simulink model "w3_warplab_trigger_proc"  (Simulink 7.7)
settings: Solver=ode45  StartTime=0.0  StopTime=60  RelTol=1e-3
InitFcn:
  | w3_warplab_trigger_proc_init
StartFcn:
  | w3_warplab_trigger_proc_init
undefined symbols (not defined in the file or in its folder): gcbh, xlBlockLoadCallback, xlGetNormalizedPeriod
libraries: xbsIndex_r4 x1289, xbsEDKLib_r4 x1, simulink x1
(part 8 of 10)

== system w3_warplab_trigger_proc/Trigger Sources/Ethernet B/Pkt Comp ==
  TVALID : Inport
  TDATA : Inport  Port=2
  TREADY : Inport  Port=3
  TLAST : Inport  Port=4
  Convert2 : xbsIndex_r4/Convert  gui_display_data_type=Boolean  arith_type=Boolean  n_bits=16  bin_pt=14  float_type=Single  exp_bits=8  fraction_bits=24  quantization=Truncate  overflow=Wrap  en=off  latency=0  dbl_ovrd=off  pipeline=off  block_type=convert
  Convert3 : xbsIndex_r4/Convert  gui_display_data_type=Boolean  arith_type=Boolean  n_bits=16  bin_pt=14  float_type=Single  exp_bits=8  fraction_bits=24  quantization=Truncate  overflow=Wrap  en=off  latency=0  dbl_ovrd=off  pipeline=off  block_type=convert
  Delay : xbsIndex_r4/Delay  rst=off  infoeditControl=Selection of Reset will increase slice count due to use of real FFs and instead of SRLs  en=off  latency=4  dbl_ovrd=off  reg_retiming=off  block_type=delay
  Delay1 : xbsIndex_r4/Delay  rst=off  infoeditControl=Selection of Reset will increase slice count due to use of real FFs and instead of SRLs  en=off  latency=3  dbl_ovrd=off  reg_retiming=off  block_type=delay
  Delay2 : xbsIndex_r4/Delay  rst=off  infoeditControl=Selection of Reset will increase slice count due to use of real FFs and instead of SRLs  en=off  latency=1  dbl_ovrd=off  reg_retiming=off  block_type=delay
  Delay3 : xbsIndex_r4/Delay  rst=off  infoeditControl=Selection of Reset will increase slice count due to use of real FFs and instead of SRLs  en=off  latency=1  dbl_ovrd=off  reg_retiming=off  block_type=delay
  Logical : xbsIndex_r4/Logical  logical_function=AND  inputs=2  en=off  latency=0  precision=Full  arith_type=Unsigned  n_bits=16  bin_pt=0  align_bp=on  dbl_ovrd=off  block_type=logical
  Output Reg 1 : Subsystem
  Pkt Match 1 : Subsystem
  Pkt Word Addr : xbsIndex_r4/Counter  cnt_type=Count Limited  cnt_to=63  operation=Up  start_count=0  cnt_by_val=1  arith_type=Unsigned  n_bits=6  bin_pt=0  load_pin=off  rst=on  en=on  explicit_period=off  period=1  dbl_ovrd=off  use_behavioral_HDL=off  implementation=Fabric  block_type=counter
  Register : xbsIndex_r4/Register  init=0  rst=off  en=off  dbl_ovrd=off  block_type=register
  Register1 : xbsIndex_r4/Register  init=0  rst=off  en=off  dbl_ovrd=off  block_type=register
  Register2 : xbsIndex_r4/Register  init=0  rst=off  en=off  dbl_ovrd=off  block_type=register
  Word Comp 1 : Subsystem
  Trigger : Outport
  wires:
  Logical/1 -> Convert2/1
  TVALID/1 -> Logical/1
  TREADY/1 -> Logical/2
  Pkt Word Addr/1 -> Word Comp 1/1(Word Addr)
  TLAST/1 -> Convert3/1
  Convert2/1 -> Pkt Word Addr/2, Delay3/1
  Convert3/1 -> Pkt Word Addr/1, Delay/1, Delay1/1
  TDATA/1 -> Delay2/1
  Delay/1 -> Register1/1
  Word Comp 1/1(Word Match) -> Pkt Match 1/2(Word Match)
  Delay1/1 -> Register2/1
  Pkt Match 1/1(Pkt Match) -> Output Reg 1/1(Match)
  Output Reg 1/1(Out) -> Trigger/1
  Delay2/1 -> Word Comp 1/2(TDATA)
  Delay3/1 -> Register/1
  Register/1 -> Pkt Match 1/1(Valid)
  Register1/1 -> Pkt Match 1/3(Reset)
  Register2/1 -> Output Reg 1/2(Done)

== system w3_warplab_trigger_proc/Trigger Sources/Energy/AntA Detector/Busy Detection ==
  Avg RSSI : Inport
  Reset : Inport  Port=2
  en : Inport  Port=3
  Convert1 : xbsIndex_r4/Convert  gui_display_data_type=Fixed-point  arith_type=Unsigned  n_bits=1  bin_pt=0  float_type=Single  exp_bits=8  fraction_bits=24  quantization=Truncate  overflow=Wrap  en=off  latency=0  dbl_ovrd=off  pipeline=off  block_type=convert
      settings: block_version=VER_STRING_GOES_HERE
  Counter1 : xbsIndex_r4/Counter  cnt_type=Free Running  cnt_to=Inf  operation=Up  start_count=0  cnt_by_val=1  arith_type=Unsigned  n_bits=11  bin_pt=0  load_pin=off  rst=on  en=on  explicit_period=off  period=4  dbl_ovrd=off  use_behavioral_HDL=off  implementation=Fabric  use_rpm=off  block_type=counter
  Display : Display
  Display1 : Display
  Gateway Out1 : xbsIndex_r4/Gateway Out  inherit_from_input=off  hdl_port=off  timing_constraint=None  locs_specified=off  LOCs={}  UseAsDAC=off  DACChannel='1'  block_type=gatewayout
  Gateway Out6 : xbsIndex_r4/Gateway Out  inherit_from_input=off  hdl_port=off  timing_constraint=None  locs_specified=off  LOCs={}  UseAsDAC=off  DACChannel='1'  block_type=gatewayout
  Inverter1 : xbsIndex_r4/Inverter  en=off  latency=0  dbl_ovrd=off  block_type=inv
      settings: xl_area=[0 0 0 0 0 0 0]  block_version=8.2
  Logical : xbsIndex_r4/Logical  logical_function=AND  inputs=2  en=off  latency=0  precision=Full  arith_type=Unsigned  n_bits=16  bin_pt=0  align_bp=on  dbl_ovrd=off  block_type=logical
  Logical1 : xbsIndex_r4/Logical  logical_function=OR  inputs=2  en=off  latency=0  precision=Full  arith_type=Unsigned  n_bits=16  bin_pt=0  align_bp=on  dbl_ovrd=off  block_type=logical
  Relational2 : xbsIndex_r4/Relational  mode=a>b  en=off  latency=0  dbl_ovrd=off  block_type=relational
      settings: block_version=VER_STRING_GOES_HERE
  Relational3 : xbsIndex_r4/Relational  mode=a>b  en=off  latency=0  dbl_ovrd=off  block_type=relational
      settings: block_version=VER_STRING_GOES_HERE
  S-R Latch : Subsystem
  Busy : Outport
  wires:
  [pktDet_energyThresh_busy] -> Relational2/2, Gateway Out6/1
  Reset/1 -> Logical1/1
  Logical1/1 -> Counter1/1, S-R Latch/1(R)
  Inverter1/1 -> Logical1/2
  Counter1/1 -> Relational3/1
  [pktDet_duration_busy] -> Relational3/2, Gateway Out1/1
  Relational3/1 -> S-R Latch/2(S)
  S-R Latch/1(Q) -> Convert1/1
  Avg RSSI/1 -> Relational2/1
  Convert1/1 -> Busy/1
  Logical/1 -> Counter1/2
  Relational2/1 -> Logical/1, Inverter1/1
  en/1 -> Logical/2
  Gateway Out6/1 -> Display/1
  Gateway Out1/1 -> Display1/1

== system w3_warplab_trigger_proc/Trigger Sources/Energy/AntA Detector/Idle Detection ==
  Avg RSSI : Inport
  Reset : Inport  Port=2
  en : Inport  Port=3
  Convert1 : xbsIndex_r4/Convert  gui_display_data_type=Fixed-point  arith_type=Unsigned  n_bits=1  bin_pt=0  float_type=Single  exp_bits=8  fraction_bits=24  quantization=Truncate  overflow=Wrap  en=off  latency=0  dbl_ovrd=off  pipeline=off  block_type=convert
      settings: block_version=VER_STRING_GOES_HERE
  Counter1 : xbsIndex_r4/Counter  cnt_type=Free Running  cnt_to=Inf  operation=Up  start_count=0  cnt_by_val=1  arith_type=Unsigned  n_bits=11  bin_pt=0  load_pin=off  rst=on  en=on  explicit_period=off  period=4  dbl_ovrd=off  use_behavioral_HDL=off  implementation=Fabric  use_rpm=off  block_type=counter
  Display : Display
  Display1 : Display
  Gateway Out1 : xbsIndex_r4/Gateway Out  inherit_from_input=off  hdl_port=off  timing_constraint=None  locs_specified=off  LOCs={}  UseAsDAC=off  DACChannel='1'  block_type=gatewayout
  Gateway Out6 : xbsIndex_r4/Gateway Out  inherit_from_input=off  hdl_port=off  timing_constraint=None  locs_specified=off  LOCs={}  UseAsDAC=off  DACChannel='1'  block_type=gatewayout
  Inverter1 : xbsIndex_r4/Inverter  en=off  latency=0  dbl_ovrd=off  block_type=inv
      settings: xl_area=[0 0 0 0 0 0 0]  block_version=8.2
  Logical : xbsIndex_r4/Logical  logical_function=AND  inputs=2  en=off  latency=0  precision=Full  arith_type=Unsigned  n_bits=16  bin_pt=0  align_bp=on  dbl_ovrd=off  block_type=logical
  Logical1 : xbsIndex_r4/Logical  logical_function=OR  inputs=2  en=off  latency=0  precision=Full  arith_type=Unsigned  n_bits=16  bin_pt=0  align_bp=on  dbl_ovrd=off  block_type=logical
  Relational2 : xbsIndex_r4/Relational  mode=a<b  en=off  latency=0  dbl_ovrd=off  block_type=relational
      settings: block_version=VER_STRING_GOES_HERE
  Relational3 : xbsIndex_r4/Relational  mode=a>b  en=off  latency=0  dbl_ovrd=off  block_type=relational
      settings: block_version=VER_STRING_GOES_HERE
  S-R Latch : Subsystem
  Idle : Outport
  wires:
  Convert1/1 -> Idle/1
  Avg RSSI/1 -> Relational2/1
  S-R Latch/1(Q) -> Convert1/1
  Relational3/1 -> S-R Latch/2(S)
  [pktDet_duration_idle] -> Relational3/2, Gateway Out1/1
  Counter1/1 -> Relational3/1
  Inverter1/1 -> Logical1/2
  Logical1/1 -> Counter1/1, S-R Latch/1(R)
  Reset/1 -> Logical1/1
  Relational2/1 -> Logical/1, Inverter1/1
  [pktDet_energyThresh_idle] -> Relational2/2, Gateway Out6/1
  en/1 -> Logical/2
  Logical/1 -> Counter1/2
  Gateway Out6/1 -> Display/1
  Gateway Out1/1 -> Display1/1

== system w3_warplab_trigger_proc/Trigger Sources/Energy/AntA Detector/Running Sum ==
  note: This block impelemnts a variable-length running sum.
      | For a sum y(n) of the previous N samples of sequence x(n), it implements
      | y(n) = y(n-1) + x(n) - x(n-N)
      | This requires a careful reset procedure, where the full shift register
      | is zerored out. Otherwise the feedback-based sum stops working.
  RSSI : Inport
  reset : Inport  Port=2
  avglen : Inport  Port=3
  en : Inport  Port=4
  ASR : xbsIndex_r4/Addressable Shift Register  infer_latency=on  depth=2  initVector=[0]  en=on  dbl_ovrd=off  use_behavioral_HDL=off  Optimization=Resource  use_rpm=off  block_type=addrsr
      settings: infoedit="Delay of configurable length.  Any element in the delay line can be addressed and driven onto the output port.<br><br>Hardware notes: This block is implemented using SRL16s. If Virtex-4 or Spartan-3 device is used, multiple SRLC16s are cascaded together."  block_version=VER_STRING_GOES_HERE
  Accumulator : xbsIndex_r4/Accumulator  operation=Add  n_bits=17  overflow=Flag as error  scale=1  rst=on  infoeditControl=reset for floating point data type must be asserted for a minimum of 2 cycles  hasbypass=off  en=on  latency=0  dbl_ovrd=off  msb_inp=100  msb=100  lsb=-100  use_behavioral_HDL=on  implementation=Fabric  block_type=accum
      settings: block_version=VER_STRING_GOES_HERE
  AddSub : xbsIndex_r4/AddSub  mode=Subtraction  use_carryin=off  use_carryout=off  en=off  latency=0  precision=Full  arith_type=Unsigned  n_bits=10  bin_pt=0  quantization=Truncate  overflow=Wrap  dbl_ovrd=off  use_behavioral_HDL=off  hw_selection=Fabric  pipelined=off  use_rpm=on  block_type=addsub
      settings: block_version=VER_STRING_GOES_HERE
  Convert7 : xbsIndex_r4/Convert  gui_display_data_type=Fixed-point  arith_type=Unsigned  n_bits=17  bin_pt=0  float_type=Single  exp_bits=8  fraction_bits=24  quantization=Truncate  overflow=Saturate  en=off  latency=0  dbl_ovrd=off  pipeline=off  block_type=convert
      settings: block_version=10.1.3
  Logical : xbsIndex_r4/Logical  logical_function=OR  inputs=2  en=off  latency=0  precision=Full  arith_type=Unsigned  n_bits=16  bin_pt=0  align_bp=on  dbl_ovrd=off  block_type=logical
  Long Reset Gen : Subsystem
  Register : xbsIndex_r4/Register  init=0  rst=on  en=off  dbl_ovrd=off  block_type=register
      settings: block_version=VER_STRING_GOES_HERE
  avg : Outport
  wires:
  ASR/1 -> AddSub/2
  AddSub/1 -> Accumulator/1
  Register/1 -> ASR/1, AddSub/1
  avglen/1 -> ASR/2, Long Reset Gen/1(duration)
  RSSI/1 -> Register/1
  Accumulator/1 -> Convert7/1
  Logical/1 -> Register/2, Accumulator/2
  reset/1 -> Long Reset Gen/2(reset_in), Logical/2
  Long Reset Gen/1(reset_out) -> Logical/1
  Convert7/1 -> avg/1
  en/1 -> ASR/3, Accumulator/3

== system w3_warplab_trigger_proc/Trigger Sources/Energy/AntB Detector/Busy Detection ==
  Avg RSSI : Inport
  Reset : Inport  Port=2
  en : Inport  Port=3
  Convert1 : xbsIndex_r4/Convert  gui_display_data_type=Fixed-point  arith_type=Unsigned  n_bits=1  bin_pt=0  float_type=Single  exp_bits=8  fraction_bits=24  quantization=Truncate  overflow=Wrap  en=off  latency=0  dbl_ovrd=off  pipeline=off  block_type=convert
      settings: block_version=VER_STRING_GOES_HERE
  Counter1 : xbsIndex_r4/Counter  cnt_type=Free Running  cnt_to=Inf  operation=Up  start_count=0  cnt_by_val=1  arith_type=Unsigned  n_bits=11  bin_pt=0  load_pin=off  rst=on  en=on  explicit_period=off  period=4  dbl_ovrd=off  use_behavioral_HDL=off  implementation=Fabric  use_rpm=off  block_type=counter
  Inverter1 : xbsIndex_r4/Inverter  en=off  latency=0  dbl_ovrd=off  block_type=inv
      settings: xl_area=[0 0 0 0 0 0 0]  block_version=8.2
  Logical : xbsIndex_r4/Logical  logical_function=AND  inputs=2  en=off  latency=0  precision=Full  arith_type=Unsigned  n_bits=16  bin_pt=0  align_bp=on  dbl_ovrd=off  block_type=logical
  Logical1 : xbsIndex_r4/Logical  logical_function=OR  inputs=2  en=off  latency=0  precision=Full  arith_type=Unsigned  n_bits=16  bin_pt=0  align_bp=on  dbl_ovrd=off  block_type=logical
  Relational2 : xbsIndex_r4/Relational  mode=a>b  en=off  latency=0  dbl_ovrd=off  block_type=relational
      settings: block_version=VER_STRING_GOES_HERE
  Relational3 : xbsIndex_r4/Relational  mode=a>b  en=off  latency=0  dbl_ovrd=off  block_type=relational
      settings: block_version=VER_STRING_GOES_HERE
  S-R Latch : Subsystem
  Busy : Outport
  wires:
  [pktDet_energyThresh_busy] -> Relational2/2
  Reset/1 -> Logical1/1
  Logical1/1 -> Counter1/1, S-R Latch/1(R)
  Inverter1/1 -> Logical1/2
  Counter1/1 -> Relational3/1
  [pktDet_duration_busy] -> Relational3/2
  Relational3/1 -> S-R Latch/2(S)
  S-R Latch/1(Q) -> Convert1/1
  Avg RSSI/1 -> Relational2/1
  Convert1/1 -> Busy/1
  Logical/1 -> Counter1/2
  Relational2/1 -> Logical/1, Inverter1/1
  en/1 -> Logical/2

== system w3_warplab_trigger_proc/Trigger Sources/Energy/AntB Detector/Idle Detection ==
  Avg RSSI : Inport
  Reset : Inport  Port=2
  en : Inport  Port=3
  Convert1 : xbsIndex_r4/Convert  gui_display_data_type=Fixed-point  arith_type=Unsigned  n_bits=1  bin_pt=0  float_type=Single  exp_bits=8  fraction_bits=24  quantization=Truncate  overflow=Wrap  en=off  latency=0  dbl_ovrd=off  pipeline=off  block_type=convert
      settings: block_version=VER_STRING_GOES_HERE
  Counter1 : xbsIndex_r4/Counter  cnt_type=Free Running  cnt_to=Inf  operation=Up  start_count=0  cnt_by_val=1  arith_type=Unsigned  n_bits=11  bin_pt=0  load_pin=off  rst=on  en=on  explicit_period=off  period=4  dbl_ovrd=off  use_behavioral_HDL=off  implementation=Fabric  use_rpm=off  block_type=counter
  Inverter1 : xbsIndex_r4/Inverter  en=off  latency=0  dbl_ovrd=off  block_type=inv
      settings: xl_area=[0 0 0 0 0 0 0]  block_version=8.2
  Logical : xbsIndex_r4/Logical  logical_function=AND  inputs=2  en=off  latency=0  precision=Full  arith_type=Unsigned  n_bits=16  bin_pt=0  align_bp=on  dbl_ovrd=off  block_type=logical
  Logical1 : xbsIndex_r4/Logical  logical_function=OR  inputs=2  en=off  latency=0  precision=Full  arith_type=Unsigned  n_bits=16  bin_pt=0  align_bp=on  dbl_ovrd=off  block_type=logical
  Relational2 : xbsIndex_r4/Relational  mode=a<b  en=off  latency=0  dbl_ovrd=off  block_type=relational
      settings: block_version=VER_STRING_GOES_HERE
  Relational3 : xbsIndex_r4/Relational  mode=a>b  en=off  latency=0  dbl_ovrd=off  block_type=relational
      settings: block_version=VER_STRING_GOES_HERE
  S-R Latch : Subsystem
  Idle : Outport
  wires:
  Convert1/1 -> Idle/1
  Avg RSSI/1 -> Relational2/1
  S-R Latch/1(Q) -> Convert1/1
  Relational3/1 -> S-R Latch/2(S)
  [pktDet_duration_idle] -> Relational3/2
  Counter1/1 -> Relational3/1
  Inverter1/1 -> Logical1/2
  Logical1/1 -> Counter1/1, S-R Latch/1(R)
  Reset/1 -> Logical1/1
  Relational2/1 -> Logical/1, Inverter1/1
  [pktDet_energyThresh_idle] -> Relational2/2
  en/1 -> Logical/2
  Logical/1 -> Counter1/2

== system w3_warplab_trigger_proc/Trigger Sources/Energy/AntB Detector/Running Sum ==
  note: This block impelemnts a variable-length running sum.
      | For a sum y(n) of the previous N samples of sequence x(n), it implements
      | y(n) = y(n-1) + x(n) - x(n-N)
      | This requires a careful reset procedure, where the full shift register
      | is zerored out. Otherwise the feedback-based sum stops working.
  RSSI : Inport
  reset : Inport  Port=2
  avglen : Inport  Port=3
  en : Inport  Port=4
  ASR : xbsIndex_r4/Addressable Shift Register  infer_latency=on  depth=2  initVector=[0]  en=on  dbl_ovrd=off  use_behavioral_HDL=off  Optimization=Resource  use_rpm=off  block_type=addrsr
      settings: infoedit="Delay of configurable length.  Any element in the delay line can be addressed and driven onto the output port.<br><br>Hardware notes: This block is implemented using SRL16s. If Virtex-4 or Spartan-3 device is used, multiple SRLC16s are cascaded together."  block_version=VER_STRING_GOES_HERE
  Accumulator : xbsIndex_r4/Accumulator  operation=Add  n_bits=17  overflow=Flag as error  scale=1  rst=on  infoeditControl=reset for floating point data type must be asserted for a minimum of 2 cycles  hasbypass=off  en=on  latency=0  dbl_ovrd=off  msb_inp=100  msb=100  lsb=-100  use_behavioral_HDL=on  implementation=Fabric  block_type=accum
      settings: block_version=VER_STRING_GOES_HERE
  AddSub : xbsIndex_r4/AddSub  mode=Subtraction  use_carryin=off  use_carryout=off  en=off  latency=0  precision=Full  arith_type=Unsigned  n_bits=10  bin_pt=0  quantization=Truncate  overflow=Wrap  dbl_ovrd=off  use_behavioral_HDL=off  hw_selection=Fabric  pipelined=off  use_rpm=on  block_type=addsub
      settings: block_version=VER_STRING_GOES_HERE
  Convert7 : xbsIndex_r4/Convert  gui_display_data_type=Fixed-point  arith_type=Unsigned  n_bits=17  bin_pt=0  float_type=Single  exp_bits=8  fraction_bits=24  quantization=Truncate  overflow=Saturate  en=off  latency=0  dbl_ovrd=off  pipeline=off  block_type=convert
      settings: block_version=10.1.3
  Logical : xbsIndex_r4/Logical  logical_function=OR  inputs=2  en=off  latency=0  precision=Full  arith_type=Unsigned  n_bits=16  bin_pt=0  align_bp=on  dbl_ovrd=off  block_type=logical
  Long Reset Gen : Subsystem
  Register : xbsIndex_r4/Register  init=0  rst=on  en=off  dbl_ovrd=off  block_type=register
      settings: block_version=VER_STRING_GOES_HERE
  avg : Outport
  wires:
  en/1 -> Accumulator/3, ASR/3
  Convert7/1 -> avg/1
  Long Reset Gen/1(reset_out) -> Logical/1
  reset/1 -> Logical/2, Long Reset Gen/2(reset_in)
  Logical/1 -> Accumulator/2, Register/2
  Accumulator/1 -> Convert7/1
  RSSI/1 -> Register/1
  avglen/1 -> Long Reset Gen/1(duration), ASR/2
  Register/1 -> AddSub/1, ASR/1
  AddSub/1 -> Accumulator/1
  ASR/1 -> AddSub/2

== system w3_warplab_trigger_proc/Trigger Sources/Energy/AntC Detector/Busy Detection ==
  Avg RSSI : Inport
  Reset : Inport  Port=2
  en : Inport  Port=3
  Convert1 : xbsIndex_r4/Convert  gui_display_data_type=Fixed-point  arith_type=Unsigned  n_bits=1  bin_pt=0  float_type=Single  exp_bits=8  fraction_bits=24  quantization=Truncate  overflow=Wrap  en=off  latency=0  dbl_ovrd=off  pipeline=off  block_type=convert
      settings: block_version=VER_STRING_GOES_HERE
  Counter1 : xbsIndex_r4/Counter  cnt_type=Free Running  cnt_to=Inf  operation=Up  start_count=0  cnt_by_val=1  arith_type=Unsigned  n_bits=11  bin_pt=0  load_pin=off  rst=on  en=on  explicit_period=off  period=4  dbl_ovrd=off  use_behavioral_HDL=off  implementation=Fabric  use_rpm=off  block_type=counter
  Inverter1 : xbsIndex_r4/Inverter  en=off  latency=0  dbl_ovrd=off  block_type=inv
      settings: xl_area=[0 0 0 0 0 0 0]  block_version=8.2
  Logical : xbsIndex_r4/Logical  logical_function=AND  inputs=2  en=off  latency=0  precision=Full  arith_type=Unsigned  n_bits=16  bin_pt=0  align_bp=on  dbl_ovrd=off  block_type=logical
  Logical1 : xbsIndex_r4/Logical  logical_function=OR  inputs=2  en=off  latency=0  precision=Full  arith_type=Unsigned  n_bits=16  bin_pt=0  align_bp=on  dbl_ovrd=off  block_type=logical
  Relational2 : xbsIndex_r4/Relational  mode=a>b  en=off  latency=0  dbl_ovrd=off  block_type=relational
      settings: block_version=VER_STRING_GOES_HERE
  Relational3 : xbsIndex_r4/Relational  mode=a>b  en=off  latency=0  dbl_ovrd=off  block_type=relational
      settings: block_version=VER_STRING_GOES_HERE
  S-R Latch : Subsystem
  Busy : Outport
  wires:
  [pktDet_energyThresh_busy] -> Relational2/2
  Reset/1 -> Logical1/1
  Logical1/1 -> Counter1/1, S-R Latch/1(R)
  Inverter1/1 -> Logical1/2
  Counter1/1 -> Relational3/1
  [pktDet_duration_busy] -> Relational3/2
  Relational3/1 -> S-R Latch/2(S)
  S-R Latch/1(Q) -> Convert1/1
  Avg RSSI/1 -> Relational2/1
  Convert1/1 -> Busy/1
  Logical/1 -> Counter1/2
  Relational2/1 -> Logical/1, Inverter1/1
  en/1 -> Logical/2

== system w3_warplab_trigger_proc/Trigger Sources/Energy/AntC Detector/Idle Detection ==
  Avg RSSI : Inport
  Reset : Inport  Port=2
  en : Inport  Port=3
  Convert1 : xbsIndex_r4/Convert  gui_display_data_type=Fixed-point  arith_type=Unsigned  n_bits=1  bin_pt=0  float_type=Single  exp_bits=8  fraction_bits=24  quantization=Truncate  overflow=Wrap  en=off  latency=0  dbl_ovrd=off  pipeline=off  block_type=convert
      settings: block_version=VER_STRING_GOES_HERE
  Counter1 : xbsIndex_r4/Counter  cnt_type=Free Running  cnt_to=Inf  operation=Up  start_count=0  cnt_by_val=1  arith_type=Unsigned  n_bits=11  bin_pt=0  load_pin=off  rst=on  en=on  explicit_period=off  period=4  dbl_ovrd=off  use_behavioral_HDL=off  implementation=Fabric  use_rpm=off  block_type=counter
  Inverter1 : xbsIndex_r4/Inverter  en=off  latency=0  dbl_ovrd=off  block_type=inv
      settings: xl_area=[0 0 0 0 0 0 0]  block_version=8.2
  Logical : xbsIndex_r4/Logical  logical_function=AND  inputs=2  en=off  latency=0  precision=Full  arith_type=Unsigned  n_bits=16  bin_pt=0  align_bp=on  dbl_ovrd=off  block_type=logical
  Logical1 : xbsIndex_r4/Logical  logical_function=OR  inputs=2  en=off  latency=0  precision=Full  arith_type=Unsigned  n_bits=16  bin_pt=0  align_bp=on  dbl_ovrd=off  block_type=logical
  Relational2 : xbsIndex_r4/Relational  mode=a<b  en=off  latency=0  dbl_ovrd=off  block_type=relational
      settings: block_version=VER_STRING_GOES_HERE
  Relational3 : xbsIndex_r4/Relational  mode=a>b  en=off  latency=0  dbl_ovrd=off  block_type=relational
      settings: block_version=VER_STRING_GOES_HERE
  S-R Latch : Subsystem
  Idle : Outport
  wires:
  Convert1/1 -> Idle/1
  Avg RSSI/1 -> Relational2/1
  S-R Latch/1(Q) -> Convert1/1
  Relational3/1 -> S-R Latch/2(S)
  [pktDet_duration_idle] -> Relational3/2
  Counter1/1 -> Relational3/1
  Inverter1/1 -> Logical1/2
  Logical1/1 -> Counter1/1, S-R Latch/1(R)
  Reset/1 -> Logical1/1
  Relational2/1 -> Logical/1, Inverter1/1
  [pktDet_energyThresh_idle] -> Relational2/2
  en/1 -> Logical/2
  Logical/1 -> Counter1/2

== system w3_warplab_trigger_proc/Trigger Sources/Energy/AntC Detector/Running Sum ==
  note: This block impelemnts a variable-length running sum.
      | For a sum y(n) of the previous N samples of sequence x(n), it implements
      | y(n) = y(n-1) + x(n) - x(n-N)
      | This requires a careful reset procedure, where the full shift register
      | is zerored out. Otherwise the feedback-based sum stops working.
  RSSI : Inport
  reset : Inport  Port=2
  avglen : Inport  Port=3
  en : Inport  Port=4
  ASR : xbsIndex_r4/Addressable Shift Register  infer_latency=on  depth=2  initVector=[0]  en=on  dbl_ovrd=off  use_behavioral_HDL=off  Optimization=Resource  use_rpm=off  block_type=addrsr
      settings: infoedit="Delay of configurable length.  Any element in the delay line can be addressed and driven onto the output port.<br><br>Hardware notes: This block is implemented using SRL16s. If Virtex-4 or Spartan-3 device is used, multiple SRLC16s are cascaded together."  block_version=VER_STRING_GOES_HERE
  Accumulator : xbsIndex_r4/Accumulator  operation=Add  n_bits=17  overflow=Flag as error  scale=1  rst=on  infoeditControl=reset for floating point data type must be asserted for a minimum of 2 cycles  hasbypass=off  en=on  latency=0  dbl_ovrd=off  msb_inp=100  msb=100  lsb=-100  use_behavioral_HDL=on  implementation=Fabric  block_type=accum
      settings: block_version=VER_STRING_GOES_HERE
  AddSub : xbsIndex_r4/AddSub  mode=Subtraction  use_carryin=off  use_carryout=off  en=off  latency=0  precision=Full  arith_type=Unsigned  n_bits=10  bin_pt=0  quantization=Truncate  overflow=Wrap  dbl_ovrd=off  use_behavioral_HDL=off  hw_selection=Fabric  pipelined=off  use_rpm=on  block_type=addsub
      settings: block_version=VER_STRING_GOES_HERE
  Convert7 : xbsIndex_r4/Convert  gui_display_data_type=Fixed-point  arith_type=Unsigned  n_bits=17  bin_pt=0  float_type=Single  exp_bits=8  fraction_bits=24  quantization=Truncate  overflow=Saturate  en=off  latency=0  dbl_ovrd=off  pipeline=off  block_type=convert
      settings: block_version=10.1.3
  Logical : xbsIndex_r4/Logical  logical_function=OR  inputs=2  en=off  latency=0  precision=Full  arith_type=Unsigned  n_bits=16  bin_pt=0  align_bp=on  dbl_ovrd=off  block_type=logical
  Long Reset Gen : Subsystem
  Register : xbsIndex_r4/Register  init=0  rst=on  en=off  dbl_ovrd=off  block_type=register
      settings: block_version=VER_STRING_GOES_HERE
  avg : Outport
  wires:
  ASR/1 -> AddSub/2
  AddSub/1 -> Accumulator/1
  Register/1 -> ASR/1, AddSub/1
  avglen/1 -> ASR/2, Long Reset Gen/1(duration)
  RSSI/1 -> Register/1
  Accumulator/1 -> Convert7/1
  Logical/1 -> Register/2, Accumulator/2
  reset/1 -> Long Reset Gen/2(reset_in), Logical/2
  Long Reset Gen/1(reset_out) -> Logical/1
  Convert7/1 -> avg/1
  en/1 -> ASR/3, Accumulator/3

== system w3_warplab_trigger_proc/Trigger Sources/Energy/AntD Detector/Busy Detection ==
  Avg RSSI : Inport
  Reset : Inport  Port=2
  en : Inport  Port=3
  Convert1 : xbsIndex_r4/Convert  gui_display_data_type=Fixed-point  arith_type=Unsigned  n_bits=1  bin_pt=0  float_type=Single  exp_bits=8  fraction_bits=24  quantization=Truncate  overflow=Wrap  en=off  latency=0  dbl_ovrd=off  pipeline=off  block_type=convert
      settings: block_version=VER_STRING_GOES_HERE
  Counter1 : xbsIndex_r4/Counter  cnt_type=Free Running  cnt_to=Inf  operation=Up  start_count=0  cnt_by_val=1  arith_type=Unsigned  n_bits=11  bin_pt=0  load_pin=off  rst=on  en=on  explicit_period=off  period=4  dbl_ovrd=off  use_behavioral_HDL=off  implementation=Fabric  use_rpm=off  block_type=counter
  Inverter1 : xbsIndex_r4/Inverter  en=off  latency=0  dbl_ovrd=off  block_type=inv
      settings: xl_area=[0 0 0 0 0 0 0]  block_version=8.2
  Logical : xbsIndex_r4/Logical  logical_function=AND  inputs=2  en=off  latency=0  precision=Full  arith_type=Unsigned  n_bits=16  bin_pt=0  align_bp=on  dbl_ovrd=off  block_type=logical
  Logical1 : xbsIndex_r4/Logical  logical_function=OR  inputs=2  en=off  latency=0  precision=Full  arith_type=Unsigned  n_bits=16  bin_pt=0  align_bp=on  dbl_ovrd=off  block_type=logical
  Relational2 : xbsIndex_r4/Relational  mode=a>b  en=off  latency=0  dbl_ovrd=off  block_type=relational
      settings: block_version=VER_STRING_GOES_HERE
  Relational3 : xbsIndex_r4/Relational  mode=a>b  en=off  latency=0  dbl_ovrd=off  block_type=relational
      settings: block_version=VER_STRING_GOES_HERE
  S-R Latch : Subsystem
  Busy : Outport
  wires:
  [pktDet_energyThresh_busy] -> Relational2/2
  Reset/1 -> Logical1/1
  Logical1/1 -> Counter1/1, S-R Latch/1(R)
  Inverter1/1 -> Logical1/2
  Counter1/1 -> Relational3/1
  [pktDet_duration_busy] -> Relational3/2
  Relational3/1 -> S-R Latch/2(S)
  S-R Latch/1(Q) -> Convert1/1
  Avg RSSI/1 -> Relational2/1
  Convert1/1 -> Busy/1
  Logical/1 -> Counter1/2
  Relational2/1 -> Logical/1, Inverter1/1
  en/1 -> Logical/2

== system w3_warplab_trigger_proc/Trigger Sources/Energy/AntD Detector/Idle Detection ==
  Avg RSSI : Inport
  Reset : Inport  Port=2
  en : Inport  Port=3
  Convert1 : xbsIndex_r4/Convert  gui_display_data_type=Fixed-point  arith_type=Unsigned  n_bits=1  bin_pt=0  float_type=Single  exp_bits=8  fraction_bits=24  quantization=Truncate  overflow=Wrap  en=off  latency=0  dbl_ovrd=off  pipeline=off  block_type=convert
      settings: block_version=VER_STRING_GOES_HERE
  Counter1 : xbsIndex_r4/Counter  cnt_type=Free Running  cnt_to=Inf  operation=Up  start_count=0  cnt_by_val=1  arith_type=Unsigned  n_bits=11  bin_pt=0  load_pin=off  rst=on  en=on  explicit_period=off  period=4  dbl_ovrd=off  use_behavioral_HDL=off  implementation=Fabric  use_rpm=off  block_type=counter
  Inverter1 : xbsIndex_r4/Inverter  en=off  latency=0  dbl_ovrd=off  block_type=inv
      settings: xl_area=[0 0 0 0 0 0 0]  block_version=8.2
  Logical : xbsIndex_r4/Logical  logical_function=AND  inputs=2  en=off  latency=0  precision=Full  arith_type=Unsigned  n_bits=16  bin_pt=0  align_bp=on  dbl_ovrd=off  block_type=logical
  Logical1 : xbsIndex_r4/Logical  logical_function=OR  inputs=2  en=off  latency=0  precision=Full  arith_type=Unsigned  n_bits=16  bin_pt=0  align_bp=on  dbl_ovrd=off  block_type=logical
  Relational2 : xbsIndex_r4/Relational  mode=a<b  en=off  latency=0  dbl_ovrd=off  block_type=relational
      settings: block_version=VER_STRING_GOES_HERE
  Relational3 : xbsIndex_r4/Relational  mode=a>b  en=off  latency=0  dbl_ovrd=off  block_type=relational
      settings: block_version=VER_STRING_GOES_HERE
  S-R Latch : Subsystem
  Idle : Outport
  wires:
  Convert1/1 -> Idle/1
  Avg RSSI/1 -> Relational2/1
  S-R Latch/1(Q) -> Convert1/1
  Relational3/1 -> S-R Latch/2(S)
  [pktDet_duration_idle] -> Relational3/2
  Counter1/1 -> Relational3/1
  Inverter1/1 -> Logical1/2
  Logical1/1 -> Counter1/1, S-R Latch/1(R)
  Reset/1 -> Logical1/1
  Relational2/1 -> Logical/1, Inverter1/1
  [pktDet_energyThresh_idle] -> Relational2/2
  en/1 -> Logical/2
  Logical/1 -> Counter1/2

== system w3_warplab_trigger_proc/Trigger Sources/Energy/AntD Detector/Running Sum ==
  note: This block impelemnts a variable-length running sum.
      | For a sum y(n) of the previous N samples of sequence x(n), it implements
      | y(n) = y(n-1) + x(n) - x(n-N)
      | This requires a careful reset procedure, where the full shift register
      | is zerored out. Otherwise the feedback-based sum stops working.
  RSSI : Inport
  reset : Inport  Port=2
  avglen : Inport  Port=3
  en : Inport  Port=4
  ASR : xbsIndex_r4/Addressable Shift Register  infer_latency=on  depth=2  initVector=[0]  en=on  dbl_ovrd=off  use_behavioral_HDL=off  Optimization=Resource  use_rpm=off  block_type=addrsr
      settings: infoedit="Delay of configurable length.  Any element in the delay line can be addressed and driven onto the output port.<br><br>Hardware notes: This block is implemented using SRL16s. If Virtex-4 or Spartan-3 device is used, multiple SRLC16s are cascaded together."  block_version=VER_STRING_GOES_HERE
  Accumulator : xbsIndex_r4/Accumulator  operation=Add  n_bits=17  overflow=Flag as error  scale=1  rst=on  infoeditControl=reset for floating point data type must be asserted for a minimum of 2 cycles  hasbypass=off  en=on  latency=0  dbl_ovrd=off  msb_inp=100  msb=100  lsb=-100  use_behavioral_HDL=on  implementation=Fabric  block_type=accum
      settings: block_version=VER_STRING_GOES_HERE
  AddSub : xbsIndex_r4/AddSub  mode=Subtraction  use_carryin=off  use_carryout=off  en=off  latency=0  precision=Full  arith_type=Unsigned  n_bits=10  bin_pt=0  quantization=Truncate  overflow=Wrap  dbl_ovrd=off  use_behavioral_HDL=off  hw_selection=Fabric  pipelined=off  use_rpm=on  block_type=addsub
      settings: block_version=VER_STRING_GOES_HERE
  Convert7 : xbsIndex_r4/Convert  gui_display_data_type=Fixed-point  arith_type=Unsigned  n_bits=17  bin_pt=0  float_type=Single  exp_bits=8  fraction_bits=24  quantization=Truncate  overflow=Saturate  en=off  latency=0  dbl_ovrd=off  pipeline=off  block_type=convert
      settings: block_version=10.1.3
  Logical : xbsIndex_r4/Logical  logical_function=OR  inputs=2  en=off  latency=0  precision=Full  arith_type=Unsigned  n_bits=16  bin_pt=0  align_bp=on  dbl_ovrd=off  block_type=logical
  Long Reset Gen : Subsystem
  Register : xbsIndex_r4/Register  init=0  rst=on  en=off  dbl_ovrd=off  block_type=register
      settings: block_version=VER_STRING_GOES_HERE
  avg : Outport
  wires:
  en/1 -> Accumulator/3, ASR/3
  Convert7/1 -> avg/1
  Long Reset Gen/1(reset_out) -> Logical/1
  reset/1 -> Logical/2, Long Reset Gen/2(reset_in)
  Logical/1 -> Accumulator/2, Register/2
  Accumulator/1 -> Convert7/1
  RSSI/1 -> Register/1
  avglen/1 -> Long Reset Gen/1(duration), ASR/2
  Register/1 -> AddSub/1, ASR/1
  AddSub/1 -> Accumulator/1
  ASR/1 -> AddSub/2

== system w3_warplab_trigger_proc/Trigger Sources/Ethernet A/Pkt Comp/Output Reg 0 ==
  Match : Inport
  Done : Inport  Port=2
  Delay2 : xbsIndex_r4/Delay  rst=off  infoeditControl=Selection of Reset will increase slice count due to use of real FFs and instead of SRLs  en=off  latency=32  dbl_ovrd=off  reg_retiming=off  block_type=delay
  Register : xbsIndex_r4/Register  init=0  rst=on  en=on  dbl_ovrd=off  block_type=register
  Out : Outport
  wires:
  Delay2/1 -> Register/2
  Register/1 -> Out/1
  Match/1 -> Register/1
  Done/1 -> Delay2/1, Register/3

== system w3_warplab_trigger_proc/Trigger Sources/Ethernet A/Pkt Comp/Pkt Match 0 ==
  Valid : Inport
  Word Match : Inport  Port=2
  Reset : Inport  Port=3
  Inverter1 : xbsIndex_r4/Inverter  en=off  latency=0  dbl_ovrd=off  block_type=inv
  Inverter2 : xbsIndex_r4/Inverter  en=off  latency=0  dbl_ovrd=off  block_type=inv
  Logical3 : xbsIndex_r4/Logical  logical_function=AND  inputs=2  en=off  latency=0  precision=Full  arith_type=Unsigned  n_bits=16  bin_pt=0  align_bp=on  dbl_ovrd=off  block_type=logical
  Pkt Match Fail : Subsystem
  Pkt Match : Outport
  wires:
  Logical3/1 -> Pkt Match Fail/1(S)
  Inverter1/1 -> Logical3/2
  Pkt Match Fail/1(Q) -> Inverter2/1
  Valid/1 -> Logical3/1
  Word Match/1 -> Inverter1/1
  Inverter2/1 -> Pkt Match/1
  Reset/1 -> Pkt Match Fail/2(R)

== system w3_warplab_trigger_proc/Trigger Sources/Ethernet A/Pkt Comp/Word Comp 0 ==
  note: No state in this block- Each word is compared
      | with zero latency. All per-packet state must
      | be maintained elsewhere.
  Word Addr : Inport
  TDATA : Inport  Port=2
  Byte Comp 0 : Subsystem
  Byte Comp 1 : Subsystem
  Byte Comp 2 : Subsystem
  Byte Comp 3 : Subsystem
  Constant1 : xbsIndex_r4/Constant  const=0  gui_display_data_type=Fixed-point  arith_type=Unsigned  n_bits=32  bin_pt=0  preci_type=Single  exp_width=8  frac_width=24  explicit_period=off  period=1  equ=P=C  opselect=C  inp2=PCIN>>17  opr=+  inp1=P  carry=CIN  dbl_ovrd=off  block_type=constant
  Constant2 : xbsIndex_r4/Constant  const=0  gui_display_data_type=Fixed-point  arith_type=Unsigned  n_bits=32  bin_pt=0  preci_type=Single  exp_width=8  frac_width=24  explicit_period=off  period=1  equ=P=C  opselect=C  inp2=PCIN>>17  opr=+  inp1=P  carry=CIN  dbl_ovrd=off  block_type=constant
  Constant3 : xbsIndex_r4/Constant  const=0  gui_display_data_type=Boolean  arith_type=Boolean  n_bits=1  bin_pt=0  preci_type=Single  exp_width=8  frac_width=24  explicit_period=off  period=1  equ=P=C  opselect=C  inp2=PCIN>>17  opr=+  inp1=P  carry=CIN  dbl_ovrd=off  block_type=constant
  Constant5 : xbsIndex_r4/Constant  const=0  gui_display_data_type=Boolean  arith_type=Boolean  n_bits=1  bin_pt=0  preci_type=Single  exp_width=8  frac_width=24  explicit_period=off  period=1  equ=P=C  opselect=C  inp2=PCIN>>17  opr=+  inp1=P  carry=CIN  dbl_ovrd=off  block_type=constant
  Logical : xbsIndex_r4/Logical  logical_function=AND  inputs=4  en=off  latency=0  precision=Full  arith_type=Unsigned  n_bits=16  bin_pt=0  align_bp=on  dbl_ovrd=off  block_type=logical
  Logical1 : xbsIndex_r4/Logical  logical_function=OR  inputs=4  en=off  latency=0  precision=Full  arith_type=Unsigned  n_bits=16  bin_pt=0  align_bp=on  dbl_ovrd=off  block_type=logical
  Logical2 : xbsIndex_r4/Logical  logical_function=AND  inputs=4  en=off  latency=0  precision=Full  arith_type=Unsigned  n_bits=16  bin_pt=0  align_bp=on  dbl_ovrd=off  block_type=logical
  Mux1 : xbsIndex_r4/Mux  inputs=2  en=off  latency=0  precision=Full  arith_type=Unsigned  n_bits=16  bin_pt=14  quantization=Truncate  overflow=Wrap  dbl_ovrd=off  block_type=mux
  Register{,1..7} (8 alike) : xbsIndex_r4/Register  init=0  rst=off  en=off  dbl_ovrd=off  block_type=register
  Shared Memory1 : xbsIndex_r4/Shared Memory  shared_memory_name='PktTemplate0'  depth=64  ownership=Locally Owned and Initialized  initVector=PKT_TEMPLATE_0  en=off  mutex=Unprotected  mode=Read and Write  write_mode=Read After Write  time_out=0  latency=1  explicit_data_type=on  gui_display_data_type=Fixed-point  arith_type=Unsigned  n_bits=32  bin_pt=0  preci_type=Single  implementation=Block RAM  use_rpm=off  block_type=shmem
      settings: AttributesFormatString=<< %<shared_memory_name> >>
  Shared Memory2 : xbsIndex_r4/Shared Memory  shared_memory_name='PktOps0'  depth=64  ownership=Locally Owned and Initialized  initVector=PKT_OPS_0  en=off  mutex=Unprotected  mode=Read and Write  write_mode=Read After Write  time_out=0  latency=1  explicit_data_type=on  gui_display_data_type=Fixed-point  arith_type=Unsigned  n_bits=32  bin_pt=0  preci_type=Single  implementation=Block RAM  use_rpm=off  block_type=shmem
      settings: AttributesFormatString=<< %<shared_memory_name> >>
  Subsystem : Subsystem
  Subsystem1 : Subsystem
  Subsystem2 : Subsystem
  Word Match : Outport
  wires:
  Constant3/1 -> Shared Memory1/3
  Constant2/1 -> Shared Memory1/2
  Word Addr/1 -> Shared Memory1/1, Shared Memory2/1
  Constant1/1 -> Shared Memory2/2
  Constant5/1 -> Shared Memory2/3
  Shared Memory2/1 -> Subsystem/1(32b)
  Shared Memory1/1 -> Subsystem1/1(32b)
  TDATA/1 -> Subsystem2/1(32b)
  Subsystem2/1(B0) -> Byte Comp 0/1(Data)
  Subsystem/1(B0) -> Byte Comp 0/2(Op)
  Subsystem1/1(B0) -> Byte Comp 0/3(Template)
  Subsystem2/2(B1) -> Byte Comp 1/1(Data)
  Subsystem/2(B1) -> Byte Comp 1/2(Op)
  Subsystem1/2(B1) -> Byte Comp 1/3(Template)
  Subsystem1/3(B2) -> Byte Comp 2/3(Template)
  Subsystem/3(B2) -> Byte Comp 2/2(Op)
  Subsystem2/3(B2) -> Byte Comp 2/1(Data)
  Subsystem2/4(B3) -> Byte Comp 3/1(Data)
  Subsystem/4(B3) -> Byte Comp 3/2(Op)
  Subsystem1/4(B3) -> Byte Comp 3/3(Template)
  Logical/1 -> Mux1/2
  Logical1/1 -> Mux1/3
  Logical2/1 -> Mux1/1
  Byte Comp 2/2(Or Op) -> Register5/1
  Byte Comp 3/2(Or Op) -> Register7/1
  Byte Comp 0/2(Or Op) -> Register1/1
  Byte Comp 1/2(Or Op) -> Register3/1
  Byte Comp 0/1(Res) -> Register/1
  Byte Comp 1/1(Res) -> Register2/1
  Byte Comp 2/1(Res) -> Register4/1
  Byte Comp 3/1(Res) -> Register6/1
  Mux1/1 -> Word Match/1
  Register/1 -> Logical/1, Logical1/1
  Register1/1 -> Logical2/1
  Register2/1 -> Logical1/2, Logical/2
  Register3/1 -> Logical2/2
  Register4/1 -> Logical/3, Logical1/3
  Register5/1 -> Logical2/3
  Register6/1 -> Logical/4, Logical1/4
  Register7/1 -> Logical2/4

== system w3_warplab_trigger_proc/Trigger Sources/Ethernet B/Pkt Comp/Output Reg 1 ==
  Match : Inport
  Done : Inport  Port=2
  Delay2 : xbsIndex_r4/Delay  rst=off  infoeditControl=Selection of Reset will increase slice count due to use of real FFs and instead of SRLs  en=off  latency=32  dbl_ovrd=off  reg_retiming=off  block_type=delay
  Register : xbsIndex_r4/Register  init=0  rst=on  en=on  dbl_ovrd=off  block_type=register
  Out : Outport
  wires:
  Delay2/1 -> Register/2
  Register/1 -> Out/1
  Match/1 -> Register/1
  Done/1 -> Delay2/1, Register/3

== system w3_warplab_trigger_proc/Trigger Sources/Ethernet B/Pkt Comp/Pkt Match 1 ==
  Valid : Inport
  Word Match : Inport  Port=2
  Reset : Inport  Port=3
  Inverter1 : xbsIndex_r4/Inverter  en=off  latency=0  dbl_ovrd=off  block_type=inv
  Inverter2 : xbsIndex_r4/Inverter  en=off  latency=0  dbl_ovrd=off  block_type=inv
  Logical3 : xbsIndex_r4/Logical  logical_function=AND  inputs=2  en=off  latency=0  precision=Full  arith_type=Unsigned  n_bits=16  bin_pt=0  align_bp=on  dbl_ovrd=off  block_type=logical
  Pkt Match Fail : Subsystem
  Pkt Match : Outport
  wires:
  Logical3/1 -> Pkt Match Fail/1(S)
  Inverter1/1 -> Logical3/2
  Pkt Match Fail/1(Q) -> Inverter2/1
  Valid/1 -> Logical3/1
  Word Match/1 -> Inverter1/1
  Inverter2/1 -> Pkt Match/1
  Reset/1 -> Pkt Match Fail/2(R)

== system w3_warplab_trigger_proc/Trigger Sources/Ethernet B/Pkt Comp/Word Comp 1 ==
  note: No state in this block- Each word is compared
      | with zero latency. All per-packet state must
      | be maintained elsewhere.
  Word Addr : Inport
  TDATA : Inport  Port=2
  Byte Comp 0 : Subsystem
  Byte Comp 1 : Subsystem
  Byte Comp 2 : Subsystem
  Byte Comp 3 : Subsystem
  Constant1 : xbsIndex_r4/Constant  const=0  gui_display_data_type=Fixed-point  arith_type=Unsigned  n_bits=32  bin_pt=0  preci_type=Single  exp_width=8  frac_width=24  explicit_period=off  period=1  equ=P=C  opselect=C  inp2=PCIN>>17  opr=+  inp1=P  carry=CIN  dbl_ovrd=off  block_type=constant
  Constant2 : xbsIndex_r4/Constant  const=0  gui_display_data_type=Fixed-point  arith_type=Unsigned  n_bits=32  bin_pt=0  preci_type=Single  exp_width=8  frac_width=24  explicit_period=off  period=1  equ=P=C  opselect=C  inp2=PCIN>>17  opr=+  inp1=P  carry=CIN  dbl_ovrd=off  block_type=constant
  Constant3 : xbsIndex_r4/Constant  const=0  gui_display_data_type=Boolean  arith_type=Boolean  n_bits=1  bin_pt=0  preci_type=Single  exp_width=8  frac_width=24  explicit_period=off  period=1  equ=P=C  opselect=C  inp2=PCIN>>17  opr=+  inp1=P  carry=CIN  dbl_ovrd=off  block_type=constant
  Constant5 : xbsIndex_r4/Constant  const=0  gui_display_data_type=Boolean  arith_type=Boolean  n_bits=1  bin_pt=0  preci_type=Single  exp_width=8  frac_width=24  explicit_period=off  period=1  equ=P=C  opselect=C  inp2=PCIN>>17  opr=+  inp1=P  carry=CIN  dbl_ovrd=off  block_type=constant
  Logical : xbsIndex_r4/Logical  logical_function=AND  inputs=4  en=off  latency=0  precision=Full  arith_type=Unsigned  n_bits=16  bin_pt=0  align_bp=on  dbl_ovrd=off  block_type=logical
  Logical1 : xbsIndex_r4/Logical  logical_function=OR  inputs=4  en=off  latency=0  precision=Full  arith_type=Unsigned  n_bits=16  bin_pt=0  align_bp=on  dbl_ovrd=off  block_type=logical
  Logical2 : xbsIndex_r4/Logical  logical_function=AND  inputs=4  en=off  latency=0  precision=Full  arith_type=Unsigned  n_bits=16  bin_pt=0  align_bp=on  dbl_ovrd=off  block_type=logical
  Mux1 : xbsIndex_r4/Mux  inputs=2  en=off  latency=0  precision=Full  arith_type=Unsigned  n_bits=16  bin_pt=14  quantization=Truncate  overflow=Wrap  dbl_ovrd=off  block_type=mux
  Register{,1..7} (8 alike) : xbsIndex_r4/Register  init=0  rst=off  en=off  dbl_ovrd=off  block_type=register
  Shared Memory1 : xbsIndex_r4/Shared Memory  shared_memory_name='PktTemplate1'  depth=64  ownership=Locally Owned and Initialized  initVector=PKT_TEMPLATE_1  en=off  mutex=Unprotected  mode=Read and Write  write_mode=Read After Write  time_out=0  latency=1  explicit_data_type=on  gui_display_data_type=Fixed-point  arith_type=Unsigned  n_bits=32  bin_pt=0  preci_type=Single  implementation=Block RAM  use_rpm=off  block_type=shmem
      settings: AttributesFormatString=<< %<shared_memory_name> >>
  Shared Memory2 : xbsIndex_r4/Shared Memory  shared_memory_name='PktOps1'  depth=64  ownership=Locally Owned and Initialized  initVector=PKT_OPS_1  en=off  mutex=Unprotected  mode=Read and Write  write_mode=Read After Write  time_out=0  latency=1  explicit_data_type=on  gui_display_data_type=Fixed-point  arith_type=Unsigned  n_bits=32  bin_pt=0  preci_type=Single  implementation=Block RAM  use_rpm=off  block_type=shmem
      settings: AttributesFormatString=<< %<shared_memory_name> >>
  Subsystem : Subsystem
  Subsystem1 : Subsystem
  Subsystem2 : Subsystem
  Word Match : Outport
  wires:
  Constant3/1 -> Shared Memory1/3
  Constant2/1 -> Shared Memory1/2
  Word Addr/1 -> Shared Memory1/1, Shared Memory2/1
  Constant1/1 -> Shared Memory2/2
  Constant5/1 -> Shared Memory2/3
  Shared Memory2/1 -> Subsystem/1(32b)
  Shared Memory1/1 -> Subsystem1/1(32b)
  TDATA/1 -> Subsystem2/1(32b)
  Subsystem2/1(B0) -> Byte Comp 0/1(Data)
  Subsystem/1(B0) -> Byte Comp 0/2(Op)
  Subsystem1/1(B0) -> Byte Comp 0/3(Template)
  Subsystem2/2(B1) -> Byte Comp 1/1(Data)
  Subsystem/2(B1) -> Byte Comp 1/2(Op)
  Subsystem1/2(B1) -> Byte Comp 1/3(Template)
  Subsystem1/3(B2) -> Byte Comp 2/3(Template)
  Subsystem/3(B2) -> Byte Comp 2/2(Op)
  Subsystem2/3(B2) -> Byte Comp 2/1(Data)
  Subsystem2/4(B3) -> Byte Comp 3/1(Data)
  Subsystem/4(B3) -> Byte Comp 3/2(Op)
  Subsystem1/4(B3) -> Byte Comp 3/3(Template)
  Logical/1 -> Mux1/2
  Logical1/1 -> Mux1/3
  Logical2/1 -> Mux1/1
  Byte Comp 2/2(Or Op) -> Register5/1
  Byte Comp 3/2(Or Op) -> Register7/1
  Byte Comp 0/2(Or Op) -> Register1/1
  Byte Comp 1/2(Or Op) -> Register3/1
  Byte Comp 0/1(Res) -> Register/1
  Byte Comp 1/1(Res) -> Register2/1
  Byte Comp 2/1(Res) -> Register4/1
  Byte Comp 3/1(Res) -> Register6/1
  Mux1/1 -> Word Match/1
  Register/1 -> Logical/1, Logical1/1
  Register1/1 -> Logical2/1
  Register2/1 -> Logical1/2, Logical/2
  Register3/1 -> Logical2/2
  Register4/1 -> Logical/3, Logical1/3
  Register5/1 -> Logical2/3
  Register6/1 -> Logical/4, Logical1/4
  Register7/1 -> Logical2/4

== system w3_warplab_trigger_proc/Trigger Sources/Energy/AntA Detector/Busy Detection/S-R Latch ==
  R : Inport
  S : Inport  Port=2
  Constant1 : xbsIndex_r4/Constant  const=1  gui_display_data_type=Fixed-point  arith_type=Boolean  n_bits=1  bin_pt=0  preci_type=Single  exp_width=8  frac_width=24  explicit_period=off  period=1  equ=P=C  opselect=C  inp2=PCIN>>17  opr=+  inp1=P  carry=CIN  dbl_ovrd=off  block_type=constant
      settings: block_version=VER_STRING_GOES_HERE
  Register2 : xbsIndex_r4/Register  init=0  rst=on  en=on  dbl_ovrd=off  block_type=register
      settings: xl_area=[1 1 0 0 0 0 0]  block_version=VER_STRING_GOES_HERE
  Q : Outport
  wires:
  Constant1/1 -> Register2/1
  R/1 -> Register2/2
  Register2/1 -> Q/1
  S/1 -> Register2/3

== system w3_warplab_trigger_proc/Trigger Sources/Energy/AntA Detector/Idle Detection/S-R Latch ==
  R : Inport
  S : Inport  Port=2
  Constant1 : xbsIndex_r4/Constant  const=1  gui_display_data_type=Fixed-point  arith_type=Boolean  n_bits=1  bin_pt=0  preci_type=Single  exp_width=8  frac_width=24  explicit_period=off  period=1  equ=P=C  opselect=C  inp2=PCIN>>17  opr=+  inp1=P  carry=CIN  dbl_ovrd=off  block_type=constant
      settings: block_version=VER_STRING_GOES_HERE
  Register2 : xbsIndex_r4/Register  init=0  rst=on  en=on  dbl_ovrd=off  block_type=register
      settings: xl_area=[1 1 0 0 0 0 0]  block_version=VER_STRING_GOES_HERE
  Q : Outport
  wires:
  S/1 -> Register2/3
  Register2/1 -> Q/1
  R/1 -> Register2/2
  Constant1/1 -> Register2/1

== system w3_warplab_trigger_proc/Trigger Sources/Energy/AntA Detector/Running Sum/Long Reset Gen ==
  duration : Inport
  reset_in : Inport  Port=2
  Counter : xbsIndex_r4/Counter  cnt_type=Free Running  cnt_to=0  operation=Up  start_count=0  cnt_by_val=1  arith_type=Unsigned  n_bits=8  bin_pt=0  load_pin=off  rst=on  en=on  explicit_period=off  period=4  dbl_ovrd=off  use_behavioral_HDL=off  implementation=Fabric  use_rpm=off  block_type=counter
      settings: block_version=VER_STRING_GOES_HERE
  Relational : xbsIndex_r4/Relational  mode=a=b  en=off  latency=0  dbl_ovrd=off  block_type=relational
      settings: block_version=VER_STRING_GOES_HERE
  S-R Latch : Subsystem
  reset_out : Outport
  wires:
  Relational/1 -> Counter/1, S-R Latch/2(R)
  Counter/1 -> Relational/1
  reset_in/1 -> S-R Latch/1(S)
  duration/1 -> Relational/2
  S-R Latch/1(Q) -> Counter/2, reset_out/1

== system w3_warplab_trigger_proc/Trigger Sources/Energy/AntB Detector/Busy Detection/S-R Latch ==
  R : Inport
  S : Inport  Port=2
  Constant1 : xbsIndex_r4/Constant  const=1  gui_display_data_type=Fixed-point  arith_type=Boolean  n_bits=1  bin_pt=0  preci_type=Single  exp_width=8  frac_width=24  explicit_period=off  period=1  equ=P=C  opselect=C  inp2=PCIN>>17  opr=+  inp1=P  carry=CIN  dbl_ovrd=off  block_type=constant
      settings: block_version=VER_STRING_GOES_HERE
  Register2 : xbsIndex_r4/Register  init=0  rst=on  en=on  dbl_ovrd=off  block_type=register
      settings: xl_area=[1 1 0 0 0 0 0]  block_version=VER_STRING_GOES_HERE
  Q : Outport
  wires:
  Constant1/1 -> Register2/1
  R/1 -> Register2/2
  Register2/1 -> Q/1
  S/1 -> Register2/3

== system w3_warplab_trigger_proc/Trigger Sources/Energy/AntB Detector/Idle Detection/S-R Latch ==
  R : Inport
  S : Inport  Port=2
  Constant1 : xbsIndex_r4/Constant  const=1  gui_display_data_type=Fixed-point  arith_type=Boolean  n_bits=1  bin_pt=0  preci_type=Single  exp_width=8  frac_width=24  explicit_period=off  period=1  equ=P=C  opselect=C  inp2=PCIN>>17  opr=+  inp1=P  carry=CIN  dbl_ovrd=off  block_type=constant
      settings: block_version=VER_STRING_GOES_HERE
  Register2 : xbsIndex_r4/Register  init=0  rst=on  en=on  dbl_ovrd=off  block_type=register
      settings: xl_area=[1 1 0 0 0 0 0]  block_version=VER_STRING_GOES_HERE
  Q : Outport
  wires:
  S/1 -> Register2/3
  Register2/1 -> Q/1
  R/1 -> Register2/2
  Constant1/1 -> Register2/1

== system w3_warplab_trigger_proc/Trigger Sources/Energy/AntB Detector/Running Sum/Long Reset Gen ==
  duration : Inport
  reset_in : Inport  Port=2
  Counter : xbsIndex_r4/Counter  cnt_type=Free Running  cnt_to=0  operation=Up  start_count=0  cnt_by_val=1  arith_type=Unsigned  n_bits=8  bin_pt=0  load_pin=off  rst=on  en=on  explicit_period=off  period=4  dbl_ovrd=off  use_behavioral_HDL=off  implementation=Fabric  use_rpm=off  block_type=counter
      settings: block_version=VER_STRING_GOES_HERE
  Relational : xbsIndex_r4/Relational  mode=a=b  en=off  latency=0  dbl_ovrd=off  block_type=relational
      settings: block_version=VER_STRING_GOES_HERE
  S-R Latch : Subsystem
  reset_out : Outport
  wires:
  S-R Latch/1(Q) -> reset_out/1, Counter/2
  duration/1 -> Relational/2
  reset_in/1 -> S-R Latch/1(S)
  Counter/1 -> Relational/1
  Relational/1 -> S-R Latch/2(R), Counter/1
